simulink model "ALL_JP360_DBW_V6_5_1103"  (R2022a)
settings: Solver=FixedStepAuto  StartTime=0.0  StopTime=inf  FixedStep=0.01  RelTol=1e-3  EnableMultiTasking=on
model workspace (MAT data in the model file):
  g = 9.8
undefined symbols (not defined in the file or in its folder): canChannel, delta_v_p, IPM_Line_C0, IPM_Line_C1, IPM_Line_C2, IPM_Line_C3, M, M_p, MRR_ObjDistX, MRR_ObjDistY, MRR_ObjFusionCamID, MRR_ObjFusionSig, MRR_ObjID, MRR_ObjRelVelX, MRR_ObjRelVelY, MRR_ObjType, MRR_ObjUpdFlg, none, obj_vaild, untracktime, V, videoinput
libraries: canfdmsglib x230, canfdlib x76, slpidlib x24, simulink x18, dspstat3 x14, ctrlSharedLib x1, simulink_extras x1, imaqlib x1, realtime_pacer_lib x1, dspvision x1, visionsinks x1
(part 9 of 55)

== system ALL_JP360_DBW_V6_5_1103/CIPV1/filter/filter speed ==
  last_vaild_objs : Inport
  MRR_ObjRelVelX : Inport  Port=2
  ego_speed : Inport  Port=3
  Add : Sum
  Constant : Constant  Value=0.5  OutDataTypeStr=single
  Constant1 : Constant  Value=-1.3  OutDataTypeStr=single
  Constant2 : Constant  Value=0  OutDataTypeStr=single
  Constant3 : Constant  Value=3.6  OutDataTypeStr=single
  Constant4 : Constant  Value=-1000  OutDataTypeStr=single
  Display : Display
  Display1 : Display
  Display2 : Display
  Divide : Product  Inputs=*/
  GreaterThan : RelationalOperator  OutDataTypeStr=boolean  RndMeth=Simplest  InputSameDT=off
  Product1 : Product
  Switch1 : Switch  Criteria=u2 > Threshold  OutMin=[0]  OutMax=[80]  SaturateOnIntegerOverflow=off  InputSameDT=off
  Switch2 : Switch  Criteria=u2 > Threshold  OutMin=[0]  OutMax=[80]  SaturateOnIntegerOverflow=off  InputSameDT=off
  filter speed objs : Outport
  wires:
  Switch1/1 -> Display/1, GreaterThan/1
  GreaterThan/1 -> Display1/1, Switch2/2
  Switch2/1 -> filter speed objs/1, Display2/1
  Product1/1 -> GreaterThan/2
  Constant1/1 -> Product1/2
  Constant2/1 -> Switch2/3
  ego_speed/1 -> Divide/1
  Constant3/1 -> Divide/2
  MRR_ObjRelVelX/1 -> [MRR_ObjRelVelX]
  [MRR_ObjRelVelX] -> Switch1/1
  last_vaild_objs/1 -> [last_vaild_objs]
  [last_vaild_objs] -> Switch1/2
  Constant4/1 -> Switch1/3
  [last_vaild_objs] -> Switch2/1
  Divide/1 -> Add/1
  Constant/1 -> Add/2
  Add/1 -> Product1/1

== system ALL_JP360_DBW_V6_5_1103/CIPV1/filter/get objs width ==
  MRR_ObjFusionCamID : Inport
  MRR_ObjFusionSig : Inport  Port=2
  last_vaild_objs : Inport  Port=3
  MRR_ObjType : Inport  Port=4
  Constant : Constant  Value=0  OutDataTypeStr=single
  Constant1 : Constant  Value=-1  OutDataTypeStr=single
  Constant2 : Constant  OutDataTypeStr=single
  GreaterThan : RelationalOperator  Operator=>  OutDataTypeStr=boolean  RndMeth=Simplest  InputSameDT=off
  Product : Product
  Product1 : Product
  Product2 : Product
  Selector : Selector  IndexMode=Zero-based  InputPortWidth=8  IndexOptions=Index vector (port)  Indices=[1 3]  OutputSizes=1
  Switch2 : Switch  Criteria=u2 > Threshold  OutMin=[0]  OutMax=[80]  SaturateOnIntegerOverflow=off  InputSameDT=off
  Terminator2 : Terminator
  ipm type hlaf width : Constant  Value=[0 0.9 1.15 0.5 0.4 0.5]
  mrr type hlaf width : Constant  Value=[0 0 0 0.4 0 0.5 0 0.9]  OutDataTypeStr=single
  objs_width : Outport
  wires:
  MRR_ObjFusionSig/1 -> Product/1
  last_vaild_objs/1 -> Product2/2, Product/2
  Product/1 -> GreaterThan/1
  Constant/1 -> GreaterThan/2
  GreaterThan/1 -> Switch2/2
  Constant1/1 -> Switch2/3
  Constant2/1 -> Switch2/1
  MRR_ObjFusionCamID/1 -> Product1/1
  Switch2/1 -> Product1/2
  mrr type hlaf width/1 -> Selector/1
  MRR_ObjType/1 -> Product2/1
  Product2/1 -> Selector/2
  Selector/1 -> objs_width/1
  ipm type hlaf width/1 -> Terminator2/1

== system ALL_JP360_DBW_V6_5_1103/DCLC1/DCLC状态机/Subsystem ==
  x : Inport
  y : Inport  Port=2
  Add : Sum
  Product : Product
  Product1 : Product
  Sqrt : Sqrt
  u : Outport
  wires:
  Sqrt/1 -> u/1
  Product1/1 -> Add/2
  y/1 -> Product1/2, Product1/1
  Product/1 -> Add/1
  Add/1 -> Sqrt/1
  x/1 -> Product/2, Product/1

== system ALL_JP360_DBW_V6_5_1103/DCLC1/DCLC状态机/Subsystem1 ==
  x : Inport
  y : Inport  Port=2
  Add : Sum
  Product : Product
  Product1 : Product
  Sqrt : Sqrt
  u : Outport
  wires:
  Sqrt/1 -> u/1
  Product1/1 -> Add/2
  y/1 -> Product1/2, Product1/1
  Product/1 -> Add/1
  Add/1 -> Sqrt/1
  x/1 -> Product/2, Product/1

== system ALL_JP360_DBW_V6_5_1103/DCLC1/DCLC状态机/Subsystem2 ==
  x : Inport
  y : Inport  Port=2
  Add : Sum
  Product : Product
  Product1 : Product
  Sqrt : Sqrt
  u : Outport
  wires:
  Sqrt/1 -> u/1
  Product1/1 -> Add/2
  y/1 -> Product1/2, Product1/1
  Product/1 -> Add/1
  Add/1 -> Sqrt/1
  x/1 -> Product/2, Product/1

== system ALL_JP360_DBW_V6_5_1103/DCLC1/DCLC状态机/Subsystem3 ==
  x : Inport
  y : Inport  Port=2
  Add : Sum
  Product : Product
  Product1 : Product
  Sqrt : Sqrt
  u : Outport
  wires:
  Sqrt/1 -> u/1
  Product1/1 -> Add/2
  y/1 -> Product1/2, Product1/1
  Product/1 -> Add/1
  Add/1 -> Sqrt/1
  x/1 -> Product/2, Product/1

== system ALL_JP360_DBW_V6_5_1103/DCLC1/DCLC状态机/Subsystem4 ==
  x : Inport
  y : Inport  Port=2
  Add : Sum
  Product : Product
  Product1 : Product
  Sqrt : Sqrt
  u : Outport
  wires:
  Sqrt/1 -> u/1
  Product1/1 -> Add/2
  y/1 -> Product1/2, Product1/1
  Product/1 -> Add/1
  Add/1 -> Sqrt/1
  x/1 -> Product/2, Product/1

== system ALL_JP360_DBW_V6_5_1103/DCLC1/DCLC状态机/Subsystem5 ==
  x : Inport
  y : Inport  Port=2
  Add : Sum
  Product : Product
  Product1 : Product
  Sqrt : Sqrt
  u : Outport
  wires:
  Sqrt/1 -> u/1
  Product1/1 -> Add/2
  y/1 -> Product1/2, Product1/1
  Product/1 -> Add/1
  Add/1 -> Sqrt/1
  x/1 -> Product/2, Product/1

== system ALL_JP360_DBW_V6_5_1103/LKA_Control/LKA_Cal/ErrorCal ==
  ABS_Vhlspd : Inport
  Ct : Inport  Port=2  OutDataTypeStr=single
  SAS_SteerWheelAngle1 : Inport  Port=3
  1-D Lookup Table : Lookup_n-D  DataSpecification=Lookup table object  LookupTableObject=predict_t  BreakpointsForDimension1=[-5:5]  Table=tanh([-5:5])  UseLastTableValue=on  InternalRulePriority=Speed  RndMeth=Simplest
      settings: InputPortMap=u0,u1
  Abs1 : Abs  OutDataTypeStr=single  SaturateOnIntegerOverflow=off
  Atan : Trigonometry  Operator=atan
  Demux : Demux
  Display : Display
  Display1 : Display
  Display2 : Display
  Gain : Gain  Gain=3.27
  LatErrCal2 : Subsystem
  Mux1 : Mux  Inputs=3
  Scope : Scope  NumInputPorts=2
  Sum : Sum  Inputs=|++
  To Workspace : ToWorkspace  VariableName=C0  SaveFormat=Structure With Time  SampleTime=-1
  To Workspace1 : ToWorkspace  VariableName=C1  SaveFormat=Structure With Time  SampleTime=-1
  To Workspace2 : ToWorkspace  VariableName=C2  SaveFormat=Structure With Time  SampleTime=-1
  To Workspace3 : ToWorkspace  VariableName=C3  SaveFormat=Structure With Time  SampleTime=-1
  To Workspace5 : ToWorkspace  VariableName=predict_time1  SaveFormat=Structure With Time  SampleTime=-1
  VehiclePosePreview1 : Subsystem
  LatErr : Outport  OutDataTypeStr=single
  err_now : Outport  Port=2
  thetar : Outport  Port=3
  wires:
  Abs1/1 -> Display1/1, 1-D Lookup Table/2
  VehiclePosePreview1/3(y1) -> Mux1/3
  LatErrCal2/1(LatErr) -> LatErr/1
  Ct/1 -> LatErrCal2/1(CenterLineCoeff), Demux/1
  Mux1/1 -> LatErrCal2/2(VehPreviewPose)
  VehiclePosePreview1/1(theta/varphi) -> Mux1/1
  VehiclePosePreview1/2(x1) -> Scope/1, Mux1/2
  SAS_SteerWheelAngle1/1 -> VehiclePosePreview1/2(SAS_SteerWheelAngle)
  Demux/4 -> To Workspace3/1
  Demux/1 -> To Workspace/1, err_now/1
  Atan/1 -> thetar/1
  Demux/2 -> Sum/1, To Workspace1/1
  Demux/3 -> Abs1/1, To Workspace2/1, Gain/1
  Gain/1 -> Sum/2
  Sum/1 -> Atan/1
  1-D Lookup Table/1 -> Display2/1, VehiclePosePreview1/3(PreviewTime), To Workspace5/1
  ABS_Vhlspd/1 -> VehiclePosePreview1/1(Input), Scope/2, Display/1, 1-D Lookup Table/1

== system ALL_JP360_DBW_V6_5_1103/LKA_Control/LKA_Cal/LKAControlerl ==
  note: 目标方向盘弧度
  ABS_VehSpd : Inport
  LatErr : Inport  Port=2  OutDataTypeStr=single
  err_now : Inport  Port=3  OutDataTypeStr=single
  Line_theta : Inport  Port=4  OutDataTypeStr=single
  steer_angle : Inport  Port=5
  LKA_status : Inport  Port=6
  2-D Lookup Table : Lookup_n-D  DataSpecification=Lookup table object  LookupTableObject=lat_calibration5  BreakpointsForDimension1=[1:3]  BreakpointsForDimension2=[1:3]  UseLastTableValue=on  InternalRulePriority=Speed  RndMeth=Simplest
      settings: InputPortMap=u0,u1
  2-D Lookup Table1 : Lookup_n-D  NumberOfTableDimensions=1  DataSpecification=Lookup table object  LookupTableObject=P_Coeff  BreakpointsForDimension1=[1:3]  BreakpointsForDimension2=[1:3]  InternalRulePriority=Speed  RndMeth=Simplest
  AngleSaftyLimitedCal : MATLAB Function  TreatAsAtomicUnit=on
  Cast To Double{1,3,5..11} (9 alike) : DataTypeConversion  OutDataTypeStr=double  SaturateOnIntegerOverflow=off  RndMeth=Floor
  Constant : Constant  Value=0  OutDataTypeStr=single
  Constant1 : Constant  Value=0.365  OutDataTypeStr=single
  Constant2 : Constant  Value=0.25  OutDataTypeStr=single
  Constant3 : Constant  Value=3.27  OutDataTypeStr=single
  Constant4 : Constant  Value=0.3  OutDataTypeStr=single
  Constant5 : Constant  Value=25  OutDataTypeStr=single
  D0 : Constant  Value=0.01  OutDataTypeStr=single
  Data Store Memory : DataStoreMemory  DataStoreName=LKA_sta  ReadBeforeWriteMsg=warning  WriteAfterWriteMsg=warning  WriteAfterReadMsg=warning  ShowAdditionalParam=off  OutDataTypeStr=int8
  Data Store Memory1 : DataStoreMemory  DataStoreName=t_ca  ReadBeforeWriteMsg=warning  WriteAfterWriteMsg=warning  WriteAfterReadMsg=warning  ShowAdditionalParam=off  OutDataTypeStr=int8
  Data Store Memory2 : DataStoreMemory  DataStoreName=sta_change  ReadBeforeWriteMsg=warning  WriteAfterWriteMsg=warning  WriteAfterReadMsg=warning  ShowAdditionalParam=off  OutDataTypeStr=int8
  Dead Zone : DeadZone  LowerValue=-0.04  UpperValue=0.04
  From3 : From  Commented=on  GotoTag=steer_rate
  Gain : Gain  Gain=1/3.6
  Gain1 : Gain  Gain=180/pi
  Gain2 : Gain  Gain=-1
  Gain3 : Gain  Gain=180/pi
  Gain4 : Gain
  I0 : Constant  Value=0  OutDataTypeStr=single
  I1 : Constant  Value=10  OutDataTypeStr=single
  MATLAB Function : MATLAB Function  TreatAsAtomicUnit=on
  MaxAy : Constant  Value=2  OutDataTypeStr=single
  Moving Average : dspstat3/Moving Average  Method=Sliding window  ForgettingFactorPort=off  SpecifyWindowLength=on  WindowLength=4  ForgettingFactor=0.9  SimulateUsing=Code generation
  Mux2 : Mux  Inputs=2
  Mux3 : Mux  Inputs=2
  Mux4 : Mux
  N0 : Constant  Value=10  OutDataTypeStr=single
  P1 : Constant  Value=0.5  OutDataTypeStr=single
  PID Controller : slpidlib/PID Controller  Controller=PID  Form=Parallel  TimeDomain=Discrete-time  UseExternalTs=off  SampleTime=-1  IntegratorMethod=Forward Euler  FilterMethod=Forward Euler  ControllerParametersSource=external  P=3.5  I=0  UseKiTs=off  D=0.5  N=10  UseFilter=on  TunerSelectOption=Transfer Function Based (PID Tuner App)  InitialConditionSource=internal  InitialConditionForIntegrator=0  InitialConditionForFilter=0  DifferentiatorICPrevScaledInput=0  ExternalReset=none  TrackingMode=off  Kt=1  LimitOutput=off  SatLimitsSource=internal  UpperSaturationLimit=10  LowerSaturationLimit=-10  LinearizeAsGain=on  AntiWindupMode=none  Kb=1  RndMeth=Convergent  PGainOutDataTypeStr=single  PProdOutDataTypeStr=single  POutMin=[]  POutMax=[]  IGainOutDataTypeStr=single  IProdOutDataTypeStr=single  IOutMin=[]  IOutMax=[]  DGainOutDataTypeStr=single  DProdOutDataTypeStr=single  DOutMin=[]  DOutMax=[]  NGainOutDataTypeStr=single  NProdOutDataTypeStr=single  NOutMin=[]  NOutMax=[]  SumOutDataTypeStr=single  SumOutMin=[]  SumOutMax=[]  SaturationOutMin=[]  SaturationOutMax=[]  PParamMin=[]  PParamMax=[]  IParamMin=[]  IParamMax=[]  DParamMin=[]  DParamMax=[]  NParamMin=[]  NParamMax=[]  KbParamMin=[]  KbParamMax=[]  KtParamMin=[]  KtParamMax=[]  KbOutMin=[]  KbOutMax=[]  KtOutMin=[]  KtOutMax=[]  IntegratorOutMin=[]  IntegratorOutMax=[]  FilterOutMin=[]  FilterOutMax=[]  SumI1OutMin=[]  SumI1OutMax=[]  SumI2OutMin=[]  SumI2OutMax=[]  SumI3OutMin=[]  SumI3OutMax=[]  SumI4OutMin=[]  SumI4OutMax=[]  SumDOutMin=[]  SumDOutMax=[]  DifferentiatorOutMin=[]  DifferentiatorOutMax=[]  FilterDiffOutCoefMin=[]  FilterDiffOutCoefMax=[]  ReciprocalOutMin=[]  ReciprocalOutMax=[]  SumDenOutMin=[]  SumDenOutMax=[]  SumNumOutMin=[]  SumNumOutMax=[]  DivideOutMin=[]  DivideOutMax=[]  UdiffTsProdOutMin=[]  UdiffTsProdOutMax=[]  NTsProdOutMin=[]  NTsProdOutMax=[]  UintegralTsProdOutMin=[]  UintegralTsProdOutMax=[]  UngainTsProdOutMin=[]  UngainTsProdOutMax=[]  IntegratorContinuousStateAttributes=''  IntegratorStateMustResolveToSignalObject=off  IntegratorRTWStateStorageClass=Auto  FilterContinuousStateAttributes=''  FilterStateMustResolveToSignalObject=off  FilterRTWStateStorageClass=Auto  ParallelPVariant=ExternalParameters  IdealPVariant=Disabled  IVariant=ExternalParameters  DVariant=ExternalParameters  IntegratorVariant=Discrete  SatVariant=Disabled  AWVariant=Passthrough  PCopyVariant=Disabled  TRVariant=Disabled  FdbkBlocksVariant=Forward  IdealPFdbkVariant=Disabled  SatFdbkVariant=Disabled  DerivativeFilterVariant=ForwardEulerFilter  NVariant=ExternalParameters  NCopyVariant=Disabled  FilterICVariant=InternalICsFilter  IntegratorICVariant=InternalICs  ExternalResetVariant=Disabled  TRSumVariant=Passthrough  SumFdbkVariant=Disabled  SumVariant=Sum_PID  TsampFilterVariant=InternalTs  TsampNgainVariant=Passthrough  TsampIntegralVariant=Passthrough  ExternalSaturationOutDataTypeStr=Inherit: Same as second input  aMode=0
  PID Controller1 : slpidlib/PID Controller  Controller=PID  Form=Parallel  TimeDomain=Discrete-time  UseExternalTs=off  SampleTime=-1  IntegratorMethod=Forward Euler  FilterMethod=Forward Euler  ControllerParametersSource=external  P=3.5  I=0  UseKiTs=off  D=0.5  N=10  UseFilter=on  TunerSelectOption=Transfer Function Based (PID Tuner App)  InitialConditionSource=internal  InitialConditionForIntegrator=0  InitialConditionForFilter=0  DifferentiatorICPrevScaledInput=0  ExternalReset=none  TrackingMode=off  Kt=1  LimitOutput=off  SatLimitsSource=internal  UpperSaturationLimit=10  LowerSaturationLimit=-10  LinearizeAsGain=on  AntiWindupMode=none  Kb=1  RndMeth=Convergent  PGainOutDataTypeStr=single  PProdOutDataTypeStr=single  POutMin=[]  POutMax=[]  IGainOutDataTypeStr=single  IProdOutDataTypeStr=single  IOutMin=[]  IOutMax=[]  DGainOutDataTypeStr=single  DProdOutDataTypeStr=single  DOutMin=[]  DOutMax=[]  NGainOutDataTypeStr=single  NProdOutDataTypeStr=single  NOutMin=[]  NOutMax=[]  SumOutDataTypeStr=single  SumOutMin=[]  SumOutMax=[]  SaturationOutMin=[]  SaturationOutMax=[]  PParamMin=[]  PParamMax=[]  IParamMin=[]  IParamMax=[]  DParamMin=[]  DParamMax=[]  NParamMin=[]  NParamMax=[]  KbParamMin=[]  KbParamMax=[]  KtParamMin=[]  KtParamMax=[]  KbOutMin=[]  KbOutMax=[]  KtOutMin=[]  KtOutMax=[]  IntegratorOutMin=[]  IntegratorOutMax=[]  FilterOutMin=[]  FilterOutMax=[]  SumI1OutMin=[]  SumI1OutMax=[]  SumI2OutMin=[]  SumI2OutMax=[]  SumI3OutMin=[]  SumI3OutMax=[]  SumI4OutMin=[]  SumI4OutMax=[]  SumDOutMin=[]  SumDOutMax=[]  DifferentiatorOutMin=[]  DifferentiatorOutMax=[]  FilterDiffOutCoefMin=[]  FilterDiffOutCoefMax=[]  ReciprocalOutMin=[]  ReciprocalOutMax=[]  SumDenOutMin=[]  SumDenOutMax=[]  SumNumOutMin=[]  SumNumOutMax=[]  DivideOutMin=[]  DivideOutMax=[]  UdiffTsProdOutMin=[]  UdiffTsProdOutMax=[]  NTsProdOutMin=[]  NTsProdOutMax=[]  UintegralTsProdOutMin=[]  UintegralTsProdOutMax=[]  UngainTsProdOutMin=[]  UngainTsProdOutMax=[]  IntegratorContinuousStateAttributes=''  IntegratorStateMustResolveToSignalObject=off  IntegratorRTWStateStorageClass=Auto  FilterContinuousStateAttributes=''  FilterStateMustResolveToSignalObject=off  FilterRTWStateStorageClass=Auto  ParallelPVariant=ExternalParameters  IdealPVariant=Disabled  IVariant=ExternalParameters  DVariant=ExternalParameters  IntegratorVariant=Discrete  SatVariant=Disabled  AWVariant=Passthrough  PCopyVariant=Disabled  TRVariant=Disabled  FdbkBlocksVariant=Forward  IdealPFdbkVariant=Disabled  SatFdbkVariant=Disabled  DerivativeFilterVariant=ForwardEulerFilter  NVariant=ExternalParameters  NCopyVariant=Disabled  FilterICVariant=InternalICsFilter  IntegratorICVariant=InternalICs  ExternalResetVariant=Disabled  TRSumVariant=Passthrough  SumFdbkVariant=Disabled  SumVariant=Sum_PID  TsampFilterVariant=InternalTs  TsampNgainVariant=Passthrough  TsampIntegralVariant=Passthrough  ExternalSaturationOutDataTypeStr=Inherit: Same as second input  aMode=0
  Product : Product
  Product2 : Product
  Product3 : Product
  Rate Limiter : RateLimiter  RisingSlewLimit=3  FallingSlewLimit=-3  SampleTimeMode=inherited
  Rate Limiter Dynamic : simulink/Discontinuities/Rate Limiter Dynamic
  Saturation : Saturate  UpperLimit=4  LowerLimit=-4
  Scope : Scope  NumInputPorts=2
  Scope1 : Scope  NumInputPorts=4
  Scope2 : Scope  NumInputPorts=2
  Scope3 : Scope  NumInputPorts=3
  Sum : Sum  Inputs=++|
  Sum3 : Sum  Inputs=++|
  Sum5 : Sum  Inputs=++|
  Terminator : Terminator
  To Workspace : ToWorkspace  VariableName=lat_err  SaveFormat=Structure With Time  SampleTime=-1
  To Workspace1 : ToWorkspace  VariableName=real_angle  SaveFormat=Structure With Time  SampleTime=-1
  To Workspace10 : ToWorkspace  VariableName=err_now  SaveFormat=Structure With Time  SampleTime=-1
  To Workspace2 : ToWorkspace  VariableName=target_angle  SaveFormat=Structure With Time  SampleTime=-1
  To Workspace3 : ToWorkspace  VariableName=tor_req  SaveFormat=Structure With Time  SampleTime=-1
  To Workspace5 : ToWorkspace  VariableName=angle_max  SaveFormat=Structure With Time  SampleTime=-1
  To Workspace6 : ToWorkspace  VariableName=vehspd  SaveFormat=Structure With Time  SampleTime=-1
  To Workspace7 : ToWorkspace  VariableName=Line_angle  SaveFormat=Structure With Time  SampleTime=-1
  To Workspace8 : ToWorkspace  VariableName=PID_angle  SaveFormat=Structure With Time  SampleTime=-1
  To Workspace9 : ToWorkspace  VariableName=angle_mux  SaveFormat=Structure With Time  SampleTime=-1
  angle : Scope
  angle_max : Scope
  control : Scope
  d_ang : Constant  OutDataTypeStr=single
  lat_err : Scope
  now_err : Scope
  output_limit : Scope
  theta_inf : Scope
  weight : Constant  Value=0.5  OutDataTypeStr=single
  weight1 : Constant  Value=0.6  OutDataTypeStr=single
  SteeringAngleCommand : Outport
  wires:
  MaxAy/1 -> AngleSaftyLimitedCal/1(a)
  Constant3/1 -> AngleSaftyLimitedCal/2(L)
  ABS_VehSpd/1 -> 2-D Lookup Table1/1, 2-D Lookup Table/1, Gain/1, [vehspd]  "车速"
  AngleSaftyLimitedCal/1(angle_limited) -> Scope2/2, Rate Limiter Dynamic/2  "before"
  Dead Zone/1 -> Saturation/1
  d_ang/1 -> AngleSaftyLimitedCal/5(w)
  Gain2/1 -> Rate Limiter Dynamic/3
  [lat_err] -> To Workspace/1, lat_err/1, Cast To Double3/1
  AngleSaftyLimitedCal/2(d_ang) -> Terminator/1
  [tar_angle] -> To Workspace2/1, Cast To Double1/1
  Cast To Double3/1 -> control/1  "err"
  Mux2/1 -> output_limit/1
  Cast To Double6/1 -> Mux2/2  "real"
  Cast To Double1/1 -> angle/1, Mux2/1  "target"
  [angle_mux] -> Cast To Double6/1
  weight/1 -> Product/1
  Sum3/1 -> [angle_mux], AngleSaftyLimitedCal/4(angle)
  Gain3/1 -> [err_angle], Product/2
  Line_theta/1 -> Gain1/1
  Gain/1 -> AngleSaftyLimitedCal/3(V)
  AngleSaftyLimitedCal/3(angle_max) -> [angle_max]
  [angle_max] -> Cast To Double5/1, To Workspace5/1
  [vehspd] -> Cast To Double7/1, To Workspace6/1
  Mux3/1 -> angle_max/1
  Cast To Double5/1 -> Mux3/2  "angle_max"
  Cast To Double7/1 -> Mux3/1  "vehspd"
  [err_angle] -> To Workspace8/1, Cast To Double8/1
  [Line_angle] -> To Workspace7/1, Cast To Double9/1
  Cast To Double8/1 -> Mux4/1  "err_angle"
  Cast To Double9/1 -> Mux4/2  "Line"
  Mux4/1 -> theta_inf/1
  [angle_mux] -> To Workspace9/1, Cast To Double10/1
  Cast To Double10/1 -> Mux4/3  "mux"
  Constant4/1 -> Product3/2
  weight1/1 -> Product2/1
  LatErr/1 -> [lat_err], Product2/2
  err_now/1 -> [err_now], Product3/1
  Sum5/1 -> Dead Zone/1
  [err_now] -> To Workspace10/1, now_err/1
  [err_now] -> Cast To Double11/1
  Cast To Double11/1 -> Mux4/4  "err"
  Gain1/1 -> PID Controller1/1, [Line_angle]
  N0/1 -> PID Controller/5
  D0/1 -> PID Controller/4
  I0/1 -> PID Controller/3
  PID Controller/1 -> Gain3/1
  Product3/1 -> Sum5/1
  Product2/1 -> Sum5/2
  Saturation/1 -> PID Controller/1
  P1/1 -> PID Controller1/2
  I1/1 -> PID Controller1/5
  Constant/1 -> PID Controller1/4, PID Controller1/3
  Rate Limiter Dynamic/1 -> Sum/2, Scope2/1  "after"
  Constant2/1 -> Sum/1
  Rate Limiter/1 -> Scope/2, [tor_req], SteeringAngleCommand/1
  Moving Average/1 -> Rate Limiter/1, Scope/1
  Gain4/1 -> Moving Average/1
  2-D Lookup Table/1 -> Gain4/1
  steer_angle/1 -> To Workspace1/1, Scope1/3  "steer_ang"
  [tor_req] -> To Workspace3/1, Scope1/4  "tor_req"
  [tar_angle] -> Scope1/2  "tar_ang"
  Sum/1 -> 2-D Lookup Table/2, [tar_angle]
  MATLAB Function/1(ang_rate) -> [steer_rate]
  LKA_status/1 -> MATLAB Function/1(LKA_status)
  [err_now] -> MATLAB Function/2(err)
  [err_now] -> Scope1/1  "err"
  Constant5/1 -> Gain2/1, Rate Limiter Dynamic/1
  2-D Lookup Table1/1 -> Scope3/3
  PID Controller1/1 -> Scope3/1, Sum3/1
  Product/1 -> Scope3/2, Sum3/2
  Constant1/1 -> PID Controller/2

== system ALL_JP360_DBW_V6_5_1103/MsgFromCAN/CCAN_ADCU_MsgFromCAN/CCAN_ADCU_ABS_Sts_0x221 ==
  CCAN_ADCU_ABS_Sts_0x221FromInData : Inport  OutDataTypeStr=Bus:CAN_FD_MESSAGE_BUS
  Bus Creator : BusCreator  Inputs=12  OutDataTypeStr=Bus:CCAN_ADCU_ABS_Sts_0x221  NonVirtualBus=on
  CAN FD Unpack : canfdmsglib/CAN FD Unpack  CANdbFile=HiFire_JPT360_CCAN_Matrix_CAN_V1.72_VP_ADCU.dbc  MsgList=(none)  MsgName=ABS_Sts_0x221  ProtocolMode=CAN FD  MsgIDType=Standard (11-bit identifier)  MsgIdentifier=545  MsgLength=8  SignalInfo={'ABS_AbsCtrlActv','39','1','BE','unsigned','Standard','0','1','0','0','1';'ABS_AbsFlgFlt','38','1','BE','unsigned','Standard','0','1','0','0','1';'ABS_EbdFlgFlt','37','1','BE','unsigned','Standard','0','1','0','0','1';'ABS_VehSpdDirection','36','1','BE','unsigned','Standard','0','1','0','0','1';'ABS_VehSpdLgt','40','12','BE','unsigned','Standard','0','0.05625','0','0','230.2875';'ABS_VehSpdLgtStatus','54','2','BE','unsigned','Standard','0','1','0','0','2';'ABS_WhlMilgFrntLe','8','16','BE','unsigned','Standard','0','1','0','0','65535';'ABS_WhlMilgFrntLeStatus','52','1','BE','unsigned','Standard','0','1','0','0','1';'ABS_WhlMilgFrntRi','24','16','BE','unsigned','Standard','0','1','0','0','65535';'ABS_WhlMilgFrntRiStatus','53','1','BE','unsigned','Standard','0','1','0','0','1';'Checksum_0x221','56','8','BE','unsigned','Standard','0','1','0','0','255';'RollingCounter_0x221','48','4','BE','unsigned','Standard','0','1','0','0','15'}  IDPort=off  TimestampPort=off  ErrorPort=off  RemotePort=off  LengthPort=off  StatusPort=off  BRSPort=off  ESIPort=off  DLCPort=off  ApplyMinMax=off
      settings: SourceProductBaseCode=XP,ME,VN  DataFormat=CANdb specified signals
  Data Type Conversion{1..4,8,10} (6 alike) : DataTypeConversion  OutDataTypeStr=boolean  SaturateOnIntegerOverflow=off  RndMeth=Floor
  Data Type Conversion11 : DataTypeConversion  OutDataTypeStr=uint8  SaturateOnIntegerOverflow=off  RndMeth=Floor
  Data Type Conversion12 : DataTypeConversion  OutDataTypeStr=int8  SaturateOnIntegerOverflow=off  RndMeth=Floor
  Data Type Conversion5 : DataTypeConversion  OutDataTypeStr=single  SaturateOnIntegerOverflow=off  RndMeth=Floor
  Data Type Conversion6 : DataTypeConversion  OutDataTypeStr=int8  SaturateOnIntegerOverflow=off  RndMeth=Floor
  Data Type Conversion7 : DataTypeConversion  OutDataTypeStr=uint16  SaturateOnIntegerOverflow=off  RndMeth=Floor
  Data Type Conversion9 : DataTypeConversion  OutDataTypeStr=uint16  SaturateOnIntegerOverflow=off  RndMeth=Floor
  CCAN_ADCU_ABS_Sts_0x221FromOutData : Outport  OutDataTypeStr=Bus:CCAN_ADCU_ABS_Sts_0x221
  wires:
  CAN FD Unpack/1 -> Data Type Conversion1/1
  CAN FD Unpack/2 -> Data Type Conversion2/1
  CAN FD Unpack/3 -> Data Type Conversion3/1
  CAN FD Unpack/4 -> Data Type Conversion4/1
  CAN FD Unpack/5 -> Data Type Conversion5/1
  CAN FD Unpack/6 -> Data Type Conversion6/1
  CAN FD Unpack/7 -> Data Type Conversion7/1
  CAN FD Unpack/8 -> Data Type Conversion8/1
  CAN FD Unpack/9 -> Data Type Conversion9/1
  CAN FD Unpack/10 -> Data Type Conversion10/1
  CAN FD Unpack/11 -> Data Type Conversion11/1
  CAN FD Unpack/12 -> Data Type Conversion12/1
  Data Type Conversion1/1 -> Bus Creator/1  "ABS_AbsCtrlActv"
  Data Type Conversion2/1 -> Bus Creator/2  "ABS_AbsFlgFlt"
  Data Type Conversion3/1 -> Bus Creator/3  "ABS_EbdFlgFlt"
  Data Type Conversion4/1 -> Bus Creator/4  "ABS_VehSpdDirection"
  Data Type Conversion5/1 -> Bus Creator/5  "ABS_VehSpdLgt"
  Data Type Conversion6/1 -> Bus Creator/6  "ABS_VehSpdLgtStatus"
  Data Type Conversion7/1 -> Bus Creator/7  "ABS_WhlMilgFrntLe"
  Data Type Conversion8/1 -> Bus Creator/8  "ABS_WhlMilgFrntLeStatus"
  Data Type Conversion9/1 -> Bus Creator/9  "ABS_WhlMilgFrntRi"
  Data Type Conversion10/1 -> Bus Creator/10  "ABS_WhlMilgFrntRiStatus"
  Data Type Conversion11/1 -> Bus Creator/11  "Checksum_0x221"
  Data Type Conversion12/1 -> Bus Creator/12  "RollingCounter_0x221"
  Bus Creator/1 -> CCAN_ADCU_ABS_Sts_0x221FromOutData/1  "CCAN_ADCU_ABS_Sts_0x221FromOutData"
  CCAN_ADCU_ABS_Sts_0x221FromInData/1 -> CAN FD Unpack/1  "CCAN_ADCU_ABS_Sts_0x221FromInData"

== system ALL_JP360_DBW_V6_5_1103/MsgFromCAN/CCAN_ADCU_MsgFromCAN/CCAN_ADCU_BSD_0x275 ==
  CCAN_ADCU_BSD_0x275FromInData : Inport  OutDataTypeStr=Bus:CAN_FD_MESSAGE_BUS
  Bus Creator : BusCreator  Inputs=24  OutDataTypeStr=Bus:CCAN_ADCU_BSD_0x275  NonVirtualBus=on
  CAN FD Unpack : canfdmsglib/CAN FD Unpack  CANdbFile=HiFire_JPT360_CCAN_Matrix_CAN_V1.72_VP_ADCU.dbc  MsgList=(none)  MsgName=BSD_0x275  ProtocolMode=CAN FD  MsgIDType=Standard (11-bit identifier)  MsgIdentifier=629  MsgLength=8  SignalInfo={'BSDLCA_OFFTelltale','31','1','BE','unsigned','Standard','0','1','0','0','1';'BSD_AutoAlignmentFlag','8','2','BE','unsigned','Standard','0','1','0','0','3';'BSD_BLIS_Active','10','2','BE','unsigned','Standard','0','1','0','0','3';'BSD_BLIS_display','12','4','BE','unsigned','Standard','0','1','0','0','15';'BSD_BSDLCA_State','28','1','BE','unsigned','Standard','0','1','0','0','1';'BSD_DOA_State','26','1','BE','unsigned','Standard','0','1','0','0','1';'BSD_DOA_warningReqLeftFront','20','2','BE','unsigned','Standard','0','1','0','0','3';'BSD_DOA_warningReqLeftRear','18','2','BE','unsigned','Standard','0','1','0','0','3';'BSD_DOA_warningReqRightFront','4','2','BE','unsigned','Standard','0','1','0','0','3';'BSD_DOA_warningReqRightRear','2','2','BE','unsigned','Standard','0','1','0','0','3';'BSD_ELKwarning_left','25','1','BE','unsigned','Standard','0','1','0','0','1';'BSD_ELKwarning_right','24','1','BE','unsigned','Standard','0','1','0','0','1';'BSD_LCA_warningReqLeft','16','2','BE','unsigned','Standard','0','1','0','0','3';'BSD_LCA_warningReqRight','0','2','BE','unsigned','Standard','0','1','0','0','3';'BSD_RCTA_State','27','1','BE','unsigned','Standard','0','1','0','0','1';'BSD_RCTA_warningReqLeft','22','2','BE','unsigned','Standard','0','1','0','0','3';'BSD_RCTA_warningReqRight','6','2','BE','unsigned','Standard','0','1','0','0','3';'BSD_RCW_State','43','1','BE','unsigned','Standard','0','1','0','0','1';'BSD_RCW_warningReq','45','2','BE','unsigned','Standard','0','1','0','0','3';'Checksum_0x275','56','8','BE','unsigned','Standard','0','1','0','0','255';'DOA_OFFTelltale','29','1','BE','unsigned','Standard','0','1','0','0','1';'RCTA_OFFTelltale','30','1','BE','unsigned','Standard','0','1','0','0','1';'RCW_OFFTelltale','44','1','BE','unsigned','Standard','0','1','0','0','1';'RollingCounter_0x275','48','4','BE','unsigned','Standard','0','1','0','0','15'}  IDPort=off  TimestampPort=off  ErrorPort=off  RemotePort=off  LengthPort=off  StatusPort=off  BRSPort=off  ESIPort=off  DLCPort=off  ApplyMinMax=off
      settings: SourceProductBaseCode=XP,ME,VN  DataFormat=CANdb specified signals
  Data Type Conversion{1,5..6,11..12,15,18,21..23} (10 alike) : DataTypeConversion  OutDataTypeStr=boolean  SaturateOnIntegerOverflow=off  RndMeth=Floor
  Data Type Conversion{2..4,7..10,13..14,16..17,19,24} (13 alike) : DataTypeConversion  OutDataTypeStr=int8  SaturateOnIntegerOverflow=off  RndMeth=Floor
  Data Type Conversion20 : DataTypeConversion  OutDataTypeStr=uint8  SaturateOnIntegerOverflow=off  RndMeth=Floor
  CCAN_ADCU_BSD_0x275FromOutData : Outport  OutDataTypeStr=Bus:CCAN_ADCU_BSD_0x275
  wires:
  CAN FD Unpack/1 -> Data Type Conversion1/1
  CAN FD Unpack/2 -> Data Type Conversion2/1
  CAN FD Unpack/3 -> Data Type Conversion3/1
  CAN FD Unpack/4 -> Data Type Conversion4/1
  CAN FD Unpack/5 -> Data Type Conversion5/1
  CAN FD Unpack/6 -> Data Type Conversion6/1
  CAN FD Unpack/7 -> Data Type Conversion7/1
  CAN FD Unpack/8 -> Data Type Conversion8/1
  CAN FD Unpack/9 -> Data Type Conversion9/1
  CAN FD Unpack/10 -> Data Type Conversion10/1
  CAN FD Unpack/11 -> Data Type Conversion11/1
  CAN FD Unpack/12 -> Data Type Conversion12/1
  CAN FD Unpack/13 -> Data Type Conversion13/1
  CAN FD Unpack/14 -> Data Type Conversion14/1
  CAN FD Unpack/15 -> Data Type Conversion15/1
  CAN FD Unpack/16 -> Data Type Conversion16/1
  CAN FD Unpack/17 -> Data Type Conversion17/1
  CAN FD Unpack/18 -> Data Type Conversion18/1
  CAN FD Unpack/19 -> Data Type Conversion19/1
  CAN FD Unpack/20 -> Data Type Conversion20/1
  CAN FD Unpack/21 -> Data Type Conversion21/1
  CAN FD Unpack/22 -> Data Type Conversion22/1
  CAN FD Unpack/23 -> Data Type Conversion23/1
  CAN FD Unpack/24 -> Data Type Conversion24/1
  Data Type Conversion1/1 -> Bus Creator/1  "BSDLCA_OFFTelltale"
  Data Type Conversion2/1 -> Bus Creator/2  "BSD_AutoAlignmentFlag"
  Data Type Conversion3/1 -> Bus Creator/3  "BSD_BLIS_Active"
  Data Type Conversion4/1 -> Bus Creator/4  "BSD_BLIS_display"
  Data Type Conversion5/1 -> Bus Creator/5  "BSD_BSDLCA_State"
  Data Type Conversion6/1 -> Bus Creator/6  "BSD_DOA_State"
  Data Type Conversion7/1 -> Bus Creator/7  "BSD_DOA_warningReqLeftFront"
  Data Type Conversion8/1 -> Bus Creator/8  "BSD_DOA_warningReqLeftRear"
  Data Type Conversion9/1 -> Bus Creator/9  "BSD_DOA_warningReqRightFront"
  Data Type Conversion10/1 -> Bus Creator/10  "BSD_DOA_warningReqRightRear"
  Data Type Conversion11/1 -> Bus Creator/11  "BSD_ELKwarning_left"
  Data Type Conversion12/1 -> Bus Creator/12  "BSD_ELKwarning_right"
  Data Type Conversion13/1 -> Bus Creator/13  "BSD_LCA_warningReqLeft"
  Data Type Conversion14/1 -> Bus Creator/14  "BSD_LCA_warningReqRight"
  Data Type Conversion15/1 -> Bus Creator/15  "BSD_RCTA_State"
  Data Type Conversion16/1 -> Bus Creator/16  "BSD_RCTA_warningReqLeft"
  Data Type Conversion17/1 -> Bus Creator/17  "BSD_RCTA_warningReqRight"
  Data Type Conversion18/1 -> Bus Creator/18  "BSD_RCW_State"
  Data Type Conversion19/1 -> Bus Creator/19  "BSD_RCW_warningReq"
  Data Type Conversion20/1 -> Bus Creator/20  "Checksum_0x275"
  Data Type Conversion21/1 -> Bus Creator/21  "DOA_OFFTelltale"
  Data Type Conversion22/1 -> Bus Creator/22  "RCTA_OFFTelltale"
  Data Type Conversion23/1 -> Bus Creator/23  "RCW_OFFTelltale"
  Data Type Conversion24/1 -> Bus Creator/24  "RollingCounter_0x275"
  Bus Creator/1 -> CCAN_ADCU_BSD_0x275FromOutData/1  "CCAN_ADCU_BSD_0x275FromOutData"
  CCAN_ADCU_BSD_0x275FromInData/1 -> CAN FD Unpack/1  "CCAN_ADCU_BSD_0x275FromInData"

== system ALL_JP360_DBW_V6_5_1103/MsgFromCAN/CCAN_ADCU_MsgFromCAN/CCAN_ADCU_EPS_Advanced_0x176 ==
  CCAN_ADCU_EPS_Advanced_0x176FromInData : Inport  OutDataTypeStr=Bus:CAN_FD_MESSAGE_BUS
  Bus Creator : BusCreator  Inputs=12  OutDataTypeStr=Bus:CCAN_ADCU_EPS_Advanced_0x176  NonVirtualBus=on
  CAN FD Unpack : canfdmsglib/CAN FD Unpack  CANdbFile=HiFire_JPT360_CCAN_Matrix_CAN_V1.72_VP_ADCU.dbc  MsgList=(none)  MsgName=EPS_Advanced_0x176  ProtocolMode=CAN FD  MsgIDType=Standard (11-bit identifier)  MsgIdentifier=374  MsgLength=8  SignalInfo={'Checksum_0x176','56','8','BE','unsigned','Standard','0','1','0','0','255';'EPS_EPSPAMInh','32','8','BE','unsigned','Standard','0','1','0','0','255';'EPS_EPSPAMSts','52','4','BE','unsigned','Standard','0','1','0','0','15';'EPS_LDWControlStatus','27','2','BE','unsigned','Standard','0','1','0','0','3';'EPS_LKAControlStatus','30','2','BE','unsigned','Standard','0','1','0','0','3';'EPS_LKAResponseTorque','17','11','BE','unsigned','Standard','0','0.01','-10.24','-10.24','10.22';'EPS_LKAResponseTorqueValid','16','1','BE','unsigned','Standard','0','1','0','0','1';'EPS_PAM_SteeringSts','29','1','BE','unsigned','Standard','0','1','0','0','1';'EPS_PwrSteeringModeSts','25','2','BE','unsigned','Standard','0','1','0','0','3';'EPS_TorsionBarTorque','13','11','BE','unsigned','Standard','0','0.01','-10.24','-10.24','10.22';'EPS_TosionBarTorqueValid','12','1','BE','unsigned','Standard','0','1','0','0','1';'RollingCounter_0x176','48','4','BE','unsigned','Standard','0','1','0','0','15'}  IDPort=off  TimestampPort=off  ErrorPort=off  RemotePort=off  LengthPort=off  StatusPort=off  BRSPort=off  ESIPort=off  DLCPort=off  ApplyMinMax=off
      settings: SourceProductBaseCode=XP,ME,VN  DataFormat=CANdb specified signals
  Data Type Conversion1 : DataTypeConversion  OutDataTypeStr=uint8  SaturateOnIntegerOverflow=off  RndMeth=Floor
  Data Type Conversion10 : DataTypeConversion  OutDataTypeStr=single  SaturateOnIntegerOverflow=off  RndMeth=Floor
  Data Type Conversion11 : DataTypeConversion  OutDataTypeStr=boolean  SaturateOnIntegerOverflow=off  RndMeth=Floor
  Data Type Conversion{3..5,9,12} (5 alike) : DataTypeConversion  OutDataTypeStr=int8  SaturateOnIntegerOverflow=off  RndMeth=Floor
  Data Type Conversion2 : DataTypeConversion  OutDataTypeStr=uint8  SaturateOnIntegerOverflow=off  RndMeth=Floor
  Data Type Conversion6 : DataTypeConversion  OutDataTypeStr=single  SaturateOnIntegerOverflow=off  RndMeth=Floor
  Data Type Conversion7 : DataTypeConversion  OutDataTypeStr=boolean  SaturateOnIntegerOverflow=off  RndMeth=Floor
  Data Type Conversion8 : DataTypeConversion  OutDataTypeStr=boolean  SaturateOnIntegerOverflow=off  RndMeth=Floor
  CCAN_ADCU_EPS_Advanced_0x176FromOutData : Outport  OutDataTypeStr=Bus:CCAN_ADCU_EPS_Advanced_0x176
  wires:
  CAN FD Unpack/1 -> Data Type Conversion1/1
  CAN FD Unpack/2 -> Data Type Conversion2/1
  CAN FD Unpack/3 -> Data Type Conversion3/1
  CAN FD Unpack/4 -> Data Type Conversion4/1
  CAN FD Unpack/5 -> Data Type Conversion5/1
  CAN FD Unpack/6 -> Data Type Conversion6/1
  CAN FD Unpack/7 -> Data Type Conversion7/1
  CAN FD Unpack/8 -> Data Type Conversion8/1
  CAN FD Unpack/9 -> Data Type Conversion9/1
  CAN FD Unpack/10 -> Data Type Conversion10/1
  CAN FD Unpack/11 -> Data Type Conversion11/1
  CAN FD Unpack/12 -> Data Type Conversion12/1
  Data Type Conversion1/1 -> Bus Creator/1  "Checksum_0x176"
  Data Type Conversion2/1 -> Bus Creator/2  "EPS_EPSPAMInh"
  Data Type Conversion3/1 -> Bus Creator/3  "EPS_EPSPAMSts"
  Data Type Conversion4/1 -> Bus Creator/4  "EPS_LDWControlStatus"
  Data Type Conversion5/1 -> Bus Creator/5  "EPS_LKAControlStatus"
  Data Type Conversion6/1 -> Bus Creator/6  "EPS_LKAResponseTorque"
  Data Type Conversion7/1 -> Bus Creator/7  "EPS_LKAResponseTorqueValid"
  Data Type Conversion8/1 -> Bus Creator/8  "EPS_PAM_SteeringSts"
  Data Type Conversion9/1 -> Bus Creator/9  "EPS_PwrSteeringModeSts"
  Data Type Conversion10/1 -> Bus Creator/10  "EPS_TorsionBarTorque"
  Data Type Conversion11/1 -> Bus Creator/11  "EPS_TosionBarTorqueValid"
  Data Type Conversion12/1 -> Bus Creator/12  "RollingCounter_0x176"
  Bus Creator/1 -> CCAN_ADCU_EPS_Advanced_0x176FromOutData/1  "CCAN_ADCU_EPS_Advanced_0x176FromOutData"
  CCAN_ADCU_EPS_Advanced_0x176FromInData/1 -> CAN FD Unpack/1  "CCAN_ADCU_EPS_Advanced_0x176FromInData"

== system ALL_JP360_DBW_V6_5_1103/MsgFromCAN/CCAN_ADCU_MsgFromCAN/CCAN_ADCU_ESP_Advanced_0x234 ==
  CCAN_ADCU_ESP_Advanced_0x234FromInData : Inport  OutDataTypeStr=Bus:CAN_FD_MESSAGE_BUS
  Bus Creator : BusCreator  Inputs=24  OutDataTypeStr=Bus:CCAN_ADCU_ESP_Advanced_0x234  NonVirtualBus=on
  CAN FD Unpack : canfdmsglib/CAN FD Unpack  CANdbFile=HiFire_JPT360_CCAN_Matrix_CAN_V1.72_VP_ADCU.dbc  MsgList=(none)  MsgName=ESP_Advanced_0x234  ProtocolMode=CAN FD  MsgIDType=Standard (11-bit identifier)  MsgIdentifier=564  MsgLength=8  SignalInfo={'Checksum_0x234','56','8','BE','unsigned','Standard','0','1','0','0','255';'ESP_ABAactive','22','1','BE','unsigned','Standard','0','1','0','0','1';'ESP_ABAavailable','21','1','BE','unsigned','Standard','0','1','0','0','1';'ESP_AEBdecActive','18','1','BE','unsigned','Standard','0','1','0','0','1';'ESP_AEBdecAvailable','17','1','BE','unsigned','Standard','0','1','0','0','1';'ESP_AWBactive','26','1','BE','unsigned','Standard','0','1','0','0','1';'ESP_AWBavailable','25','1','BE','unsigned','Standard','0','1','0','0','1';'ESP_BrkFricTqTotAtWhl','40','14','BE','unsigned','Standard','0','1','0','0','10230';'ESP_BrkFricTqTotAtWhlvaild','16','1','BE','unsigned','Standard','0','1','0','0','1';'ESP_CDDActive','8','1','BE','unsigned','Standard','0','1','0','0','1';'ESP_CDDAvailable','23','1','BE','unsigned','Standard','0','1','0','0','1';'ESP_CDD_APAactive','9','1','BE','unsigned','Standard','0','1','0','0','1';'ESP_CDDerror','39','1','BE','unsigned','Standard','0','1','0','0','1';'ESP_DTCactive','24','1','BE','unsigned','Standard','0','1','0','0','1';'ESP_EBDActive','1','1','BE','unsigned','Standard','0','1','0','0','1';'ESP_ECDTempOff','14','1','BE','unsigned','Standard','0','1','0','0','1';'ESP_HBBActive','54','1','BE','unsigned','Standard','0','1','0','0','1';'ESP_NoBrakeForce','15','1','BE','unsigned','Standard','0','1','0','0','1';'ESP_PrefillActive','20','1','BE','unsigned','Standard','0','1','0','0','1';'ESP_PrefillAvailable','19','1','BE','unsigned','Standard','0','1','0','0','1';'ESP_VAMActive','55','1','BE','unsigned','Standard','0','1','0','0','1';'ESP_VDCActive','0','1','BE','unsigned','Standard','0','1','0','0','1';'ESP_VLCerror','38','1','BE','unsigned','Standard','0','1','0','0','1';'RollingCounter_0x234','48','4','BE','unsigned','Standard','0','1','0','0','15'}  IDPort=off  TimestampPort=off  ErrorPort=off  RemotePort=off  LengthPort=off  StatusPort=off  BRSPort=off  ESIPort=off  DLCPort=off  ApplyMinMax=off
      settings: SourceProductBaseCode=XP,ME,VN  DataFormat=CANdb specified signals
  Data Type Conversion1 : DataTypeConversion  OutDataTypeStr=uint8  SaturateOnIntegerOverflow=off  RndMeth=Floor
  Data Type Conversion{2..7,9..23} (21 alike) : DataTypeConversion  OutDataTypeStr=boolean  SaturateOnIntegerOverflow=off  RndMeth=Floor
  Data Type Conversion24 : DataTypeConversion  OutDataTypeStr=int8  SaturateOnIntegerOverflow=off  RndMeth=Floor
  Data Type Conversion8 : DataTypeConversion  OutDataTypeStr=int16  SaturateOnIntegerOverflow=off  RndMeth=Floor
  CCAN_ADCU_ESP_Advanced_0x234FromOutData : Outport  OutDataTypeStr=Bus:CCAN_ADCU_ESP_Advanced_0x234
  wires:
  CAN FD Unpack/1 -> Data Type Conversion1/1
  CAN FD Unpack/2 -> Data Type Conversion2/1
  CAN FD Unpack/3 -> Data Type Conversion3/1
  CAN FD Unpack/4 -> Data Type Conversion4/1
  CAN FD Unpack/5 -> Data Type Conversion5/1
  CAN FD Unpack/6 -> Data Type Conversion6/1
  CAN FD Unpack/7 -> Data Type Conversion7/1
  CAN FD Unpack/8 -> Data Type Conversion8/1
  CAN FD Unpack/9 -> Data Type Conversion9/1
  CAN FD Unpack/10 -> Data Type Conversion10/1
  CAN FD Unpack/11 -> Data Type Conversion11/1
  CAN FD Unpack/12 -> Data Type Conversion12/1
  CAN FD Unpack/13 -> Data Type Conversion13/1
  CAN FD Unpack/14 -> Data Type Conversion14/1
  CAN FD Unpack/15 -> Data Type Conversion15/1
  CAN FD Unpack/16 -> Data Type Conversion16/1
  CAN FD Unpack/17 -> Data Type Conversion17/1
  CAN FD Unpack/18 -> Data Type Conversion18/1
  CAN FD Unpack/19 -> Data Type Conversion19/1
  CAN FD Unpack/20 -> Data Type Conversion20/1
  CAN FD Unpack/21 -> Data Type Conversion21/1
  CAN FD Unpack/22 -> Data Type Conversion22/1
  CAN FD Unpack/23 -> Data Type Conversion23/1
  CAN FD Unpack/24 -> Data Type Conversion24/1
  Data Type Conversion1/1 -> Bus Creator/1  "Checksum_0x234"
  Data Type Conversion2/1 -> Bus Creator/2  "ESP_ABAactive"
  Data Type Conversion3/1 -> Bus Creator/3  "ESP_ABAavailable"
  Data Type Conversion4/1 -> Bus Creator/4  "ESP_AEBdecActive"
  Data Type Conversion5/1 -> Bus Creator/5  "ESP_AEBdecAvailable"
  Data Type Conversion6/1 -> Bus Creator/6  "ESP_AWBactive"
  Data Type Conversion7/1 -> Bus Creator/7  "ESP_AWBavailable"
  Data Type Conversion8/1 -> Bus Creator/8  "ESP_BrkFricTqTotAtWhl"
  Data Type Conversion9/1 -> Bus Creator/9  "ESP_BrkFricTqTotAtWhlvaild"
  Data Type Conversion10/1 -> Bus Creator/10  "ESP_CDDActive"
  Data Type Conversion11/1 -> Bus Creator/11  "ESP_CDDAvailable"
  Data Type Conversion12/1 -> Bus Creator/12  "ESP_CDD_APAactive"
  Data Type Conversion13/1 -> Bus Creator/13  "ESP_CDDerror"
  Data Type Conversion14/1 -> Bus Creator/14  "ESP_DTCactive"
  Data Type Conversion15/1 -> Bus Creator/15  "ESP_EBDActive"
  Data Type Conversion16/1 -> Bus Creator/16  "ESP_ECDTempOff"
  Data Type Conversion17/1 -> Bus Creator/17  "ESP_HBBActive"
  Data Type Conversion18/1 -> Bus Creator/18  "ESP_NoBrakeForce"
  Data Type Conversion19/1 -> Bus Creator/19  "ESP_PrefillActive"
  Data Type Conversion20/1 -> Bus Creator/20  "ESP_PrefillAvailable"
  Data Type Conversion21/1 -> Bus Creator/21  "ESP_VAMActive"
  Data Type Conversion22/1 -> Bus Creator/22  "ESP_VDCActive"
  Data Type Conversion23/1 -> Bus Creator/23  "ESP_VLCerror"
  Data Type Conversion24/1 -> Bus Creator/24  "RollingCounter_0x234"
  Bus Creator/1 -> CCAN_ADCU_ESP_Advanced_0x234FromOutData/1  "CCAN_ADCU_ESP_Advanced_0x234FromOutData"
  CCAN_ADCU_ESP_Advanced_0x234FromInData/1 -> CAN FD Unpack/1  "CCAN_ADCU_ESP_Advanced_0x234FromInData"

== system ALL_JP360_DBW_V6_5_1103/MsgFromCAN/CCAN_ADCU_MsgFromCAN/CCAN_ADCU_ESP_AxAy_0x242 ==
  CCAN_ADCU_ESP_AxAy_0x242FromInData : Inport  OutDataTypeStr=Bus:CAN_FD_MESSAGE_BUS
  Bus Creator : BusCreator  Inputs=8  OutDataTypeStr=Bus:CCAN_ADCU_ESP_AxAy_0x242  NonVirtualBus=on
  CAN FD Unpack : canfdmsglib/CAN FD Unpack  CANdbFile=HiFire_JPT360_CCAN_Matrix_CAN_V1.72_VP_ADCU.dbc  MsgList=(none)  MsgName=ESP_AxAy_0x242  ProtocolMode=CAN FD  MsgIDType=Standard (11-bit identifier)  MsgIdentifier=578  MsgLength=8  SignalInfo={'Checksum_0x242','56','8','BE','unsigned','Standard','0','1','0','0','255';'ESP_Alat','16','12','BE','unsigned','Standard','0','0.027127','-21.5931','-21.5931','21.5931';'ESP_AlatStatus','54','1','BE','unsigned','Standard','0','1','0','0','1';'ESP_Algt','12','12','BE','unsigned','Standard','0','0.027127','-21.5931','-21.5931','21.5931';'ESP_AlgtStatus','55','1','BE','unsigned','Standard','0','1','0','0','1';'ESP_YawRate','36','12','BE','unsigned','Standard','0','0.001745','-2.0942','-2.0942','5.0498';'ESP_YawRateStatus','53','1','BE','unsigned','Standard','0','1','0','0','1';'RollingCounter_0x242','48','4','BE','unsigned','Standard','0','1','0','0','15'}  IDPort=off  TimestampPort=off  ErrorPort=off  RemotePort=off  LengthPort=off  StatusPort=off  BRSPort=off  ESIPort=off  DLCPort=off  ApplyMinMax=off
      settings: SourceProductBaseCode=XP,ME,VN  DataFormat=CANdb specified signals
  Data Type Conversion1 : DataTypeConversion  OutDataTypeStr=uint8  SaturateOnIntegerOverflow=off  RndMeth=Floor
  Data Type Conversion2 : DataTypeConversion  OutDataTypeStr=single  SaturateOnIntegerOverflow=off  RndMeth=Floor
  Data Type Conversion3 : DataTypeConversion  OutDataTypeStr=boolean  SaturateOnIntegerOverflow=off  RndMeth=Floor
  Data Type Conversion4 : DataTypeConversion  OutDataTypeStr=single  SaturateOnIntegerOverflow=off  RndMeth=Floor
  Data Type Conversion5 : DataTypeConversion  OutDataTypeStr=boolean  SaturateOnIntegerOverflow=off  RndMeth=Floor
  Data Type Conversion6 : DataTypeConversion  OutDataTypeStr=single  SaturateOnIntegerOverflow=off  RndMeth=Floor
  Data Type Conversion7 : DataTypeConversion  OutDataTypeStr=boolean  SaturateOnIntegerOverflow=off  RndMeth=Floor
  Data Type Conversion8 : DataTypeConversion  OutDataTypeStr=int8  SaturateOnIntegerOverflow=off  RndMeth=Floor
  CCAN_ADCU_ESP_AxAy_0x242FromOutData : Outport  OutDataTypeStr=Bus:CCAN_ADCU_ESP_AxAy_0x242
  wires:
  CAN FD Unpack/1 -> Data Type Conversion1/1
  CAN FD Unpack/2 -> Data Type Conversion2/1
  CAN FD Unpack/3 -> Data Type Conversion3/1
  CAN FD Unpack/4 -> Data Type Conversion4/1
  CAN FD Unpack/5 -> Data Type Conversion5/1
  CAN FD Unpack/6 -> Data Type Conversion6/1
  CAN FD Unpack/7 -> Data Type Conversion7/1
  CAN FD Unpack/8 -> Data Type Conversion8/1
  Data Type Conversion1/1 -> Bus Creator/1  "Checksum_0x242"
  Data Type Conversion2/1 -> Bus Creator/2  "ESP_Alat"
  Data Type Conversion3/1 -> Bus Creator/3  "ESP_AlatStatus"
  Data Type Conversion4/1 -> Bus Creator/4  "ESP_Algt"
  Data Type Conversion5/1 -> Bus Creator/5  "ESP_AlgtStatus"
  Data Type Conversion6/1 -> Bus Creator/6  "ESP_YawRate"
  Data Type Conversion7/1 -> Bus Creator/7  "ESP_YawRateStatus"
  Data Type Conversion8/1 -> Bus Creator/8  "RollingCounter_0x242"
  Bus Creator/1 -> CCAN_ADCU_ESP_AxAy_0x242FromOutData/1  "CCAN_ADCU_ESP_AxAy_0x242FromOutData"
  CCAN_ADCU_ESP_AxAy_0x242FromInData/1 -> CAN FD Unpack/1  "CCAN_ADCU_ESP_AxAy_0x242FromInData"

== system ALL_JP360_DBW_V6_5_1103/MsgFromCAN/CCAN_ADCU_MsgFromCAN/CCAN_ADCU_ESP_Direction_0x235 ==
  CCAN_ADCU_ESP_Direction_0x235FromInData : Inport  OutDataTypeStr=Bus:CAN_FD_MESSAGE_BUS
  Bus Creator : BusCreator  Inputs=15  OutDataTypeStr=Bus:CCAN_ADCU_ESP_Direction_0x235  NonVirtualBus=on
  CAN FD Unpack : canfdmsglib/CAN FD Unpack  CANdbFile=HiFire_JPT360_CCAN_Matrix_CAN_V1.72_VP_ADCU.dbc  MsgList=(none)  MsgName=ESP_Direction_0x235  ProtocolMode=CAN FD  MsgIDType=Standard (11-bit identifier)  MsgIdentifier=565  MsgLength=8  SignalInfo={'Checksum_0x235','56','8','BE','unsigned','Standard','0','1','0','0','255';'ESP_FLWheelDriveDirStatus','33','1','BE','unsigned','Standard','0','1','0','0','1';'ESP_FLWheelDriveDirection','46','2','BE','unsigned','Standard','0','1','0','0','3';'ESP_FRWheelDriveDirStatus','32','1','BE','unsigned','Standard','0','1','0','0','1';'ESP_FRWheelDriveDirection','44','2','BE','unsigned','Standard','0','1','0','0','3';'ESP_RLWheelDriveDirStatus','35','1','BE','unsigned','Standard','0','1','0','0','1';'ESP_RLWheelDriveDirection','42','2','BE','unsigned','Standard','0','1','0','0','3';'ESP_RRWheelDriveDirStatus','34','1','BE','unsigned','Standard','0','1','0','0','1';'ESP_RRWheelDriveDirection','40','2','BE','unsigned','Standard','0','1','0','0','3';'ESP_VehicleStandstill','54','2','BE','unsigned','Standard','0','1','0','0','3';'ESP_WhlMilgReaRLeStatus','52','1','BE','unsigned','Standard','0','1','0','0','1';'ESP_WhlMilgReaRRiStatus','53','1','BE','unsigned','Standard','0','1','0','0','1';'ESP_WhlMilgRearLe','8','16','BE','unsigned','Standard','0','1','0','0','65535';'ESP_WhlMilgRearRe','24','16','BE','unsigned','Standard','0','1','0','0','65535';'RollingCounter_0x235','48','4','BE','unsigned','Standard','0','1','0','0','15'}  IDPort=off  TimestampPort=off  ErrorPort=off  RemotePort=off  LengthPort=off  StatusPort=off  BRSPort=off  ESIPort=off  DLCPort=off  ApplyMinMax=off
      settings: SourceProductBaseCode=XP,ME,VN  DataFormat=CANdb specified signals
  Data Type Conversion1 : DataTypeConversion  OutDataTypeStr=uint8  SaturateOnIntegerOverflow=off  RndMeth=Floor
  Data Type Conversion{3,5,7,9..10,15} (6 alike) : DataTypeConversion  OutDataTypeStr=int8  SaturateOnIntegerOverflow=off  RndMeth=Floor
  Data Type Conversion{2,4,6,8,11..12} (6 alike) : DataTypeConversion  OutDataTypeStr=boolean  SaturateOnIntegerOverflow=off  RndMeth=Floor
  Data Type Conversion13 : DataTypeConversion  OutDataTypeStr=uint16  SaturateOnIntegerOverflow=off  RndMeth=Floor
  Data Type Conversion14 : DataTypeConversion  OutDataTypeStr=uint16  SaturateOnIntegerOverflow=off  RndMeth=Floor
  CCAN_ADCU_ESP_Direction_0x235FromOutData : Outport  OutDataTypeStr=Bus:CCAN_ADCU_ESP_Direction_0x235
  wires:
  CAN FD Unpack/1 -> Data Type Conversion1/1
  CAN FD Unpack/2 -> Data Type Conversion2/1
  CAN FD Unpack/3 -> Data Type Conversion3/1
  CAN FD Unpack/4 -> Data Type Conversion4/1
  CAN FD Unpack/5 -> Data Type Conversion5/1
  CAN FD Unpack/6 -> Data Type Conversion6/1
  CAN FD Unpack/7 -> Data Type Conversion7/1
  CAN FD Unpack/8 -> Data Type Conversion8/1
  CAN FD Unpack/9 -> Data Type Conversion9/1
  CAN FD Unpack/10 -> Data Type Conversion10/1
  CAN FD Unpack/11 -> Data Type Conversion11/1
  CAN FD Unpack/12 -> Data Type Conversion12/1
  CAN FD Unpack/13 -> Data Type Conversion13/1
  CAN FD Unpack/14 -> Data Type Conversion14/1
  CAN FD Unpack/15 -> Data Type Conversion15/1
  Data Type Conversion1/1 -> Bus Creator/1  "Checksum_0x235"
  Data Type Conversion2/1 -> Bus Creator/2  "ESP_FLWheelDriveDirStatus"
  Data Type Conversion3/1 -> Bus Creator/3  "ESP_FLWheelDriveDirection"
  Data Type Conversion4/1 -> Bus Creator/4  "ESP_FRWheelDriveDirStatus"
  Data Type Conversion5/1 -> Bus Creator/5  "ESP_FRWheelDriveDirection"
  Data Type Conversion6/1 -> Bus Creator/6  "ESP_RLWheelDriveDirStatus"
  Data Type Conversion7/1 -> Bus Creator/7  "ESP_RLWheelDriveDirection"
  Data Type Conversion8/1 -> Bus Creator/8  "ESP_RRWheelDriveDirStatus"
  Data Type Conversion9/1 -> Bus Creator/9  "ESP_RRWheelDriveDirection"
  Data Type Conversion10/1 -> Bus Creator/10  "ESP_VehicleStandstill"
  Data Type Conversion11/1 -> Bus Creator/11  "ESP_WhlMilgReaRLeStatus"
  Data Type Conversion12/1 -> Bus Creator/12  "ESP_WhlMilgReaRRiStatus"
  Data Type Conversion13/1 -> Bus Creator/13  "ESP_WhlMilgRearLe"
  Data Type Conversion14/1 -> Bus Creator/14  "ESP_WhlMilgRearRe"
  Data Type Conversion15/1 -> Bus Creator/15  "RollingCounter_0x235"
  Bus Creator/1 -> CCAN_ADCU_ESP_Direction_0x235FromOutData/1  "CCAN_ADCU_ESP_Direction_0x235FromOutData"
  CCAN_ADCU_ESP_Direction_0x235FromInData/1 -> CAN FD Unpack/1  "CCAN_ADCU_ESP_Direction_0x235FromInData"
